simulink model "A4D_LQR_backup"  (R2016a)
settings: Solver=VariableStepAuto  StartTime=0.0  StopTime=10  RelTol=1e-3
undefined symbols (not defined in the file): A, B, C, K
settings Model: Creator=kumabhi  LastModifiedBy=kumabhi

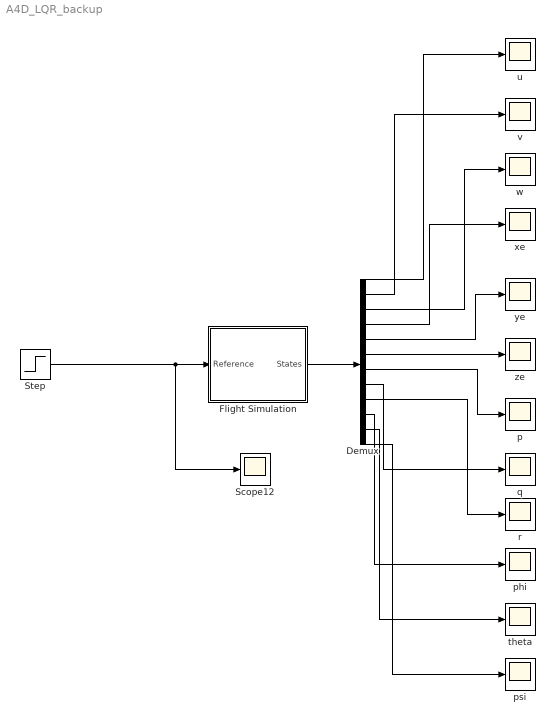
== system A4D_LQR_backup ==
  Demux : Demux  Outputs=12
  Flight Simulation : Subsystem
      mask Display: image('/home/kumabhi/Documents/Courses/Thesis/plane-icon-vector-.jpg');
  Scope12 : Scope
  Step : Step  After=1.0472  SampleTime=0
  p : Scope
  phi : Scope
  psi : Scope
  q : Scope
  r : Scope
  theta : Scope
  u : Scope
  v : Scope
  w : Scope
  xe : Scope
  ye : Scope
  ze : Scope
  wires:
  Step/1 -> Scope12/1, Flight Simulation/1(Reference)
  Flight Simulation/1(States) -> Demux/1
  Demux/1 -> u/1
  Demux/2 -> v/1
  Demux/3 -> w/1
  Demux/4 -> xe/1
  Demux/5 -> ye/1
  Demux/6 -> ze/1
  Demux/7 -> p/1
  Demux/8 -> q/1
  Demux/9 -> r/1
  Demux/10 -> phi/1
  Demux/11 -> theta/1
  Demux/12 -> psi/1

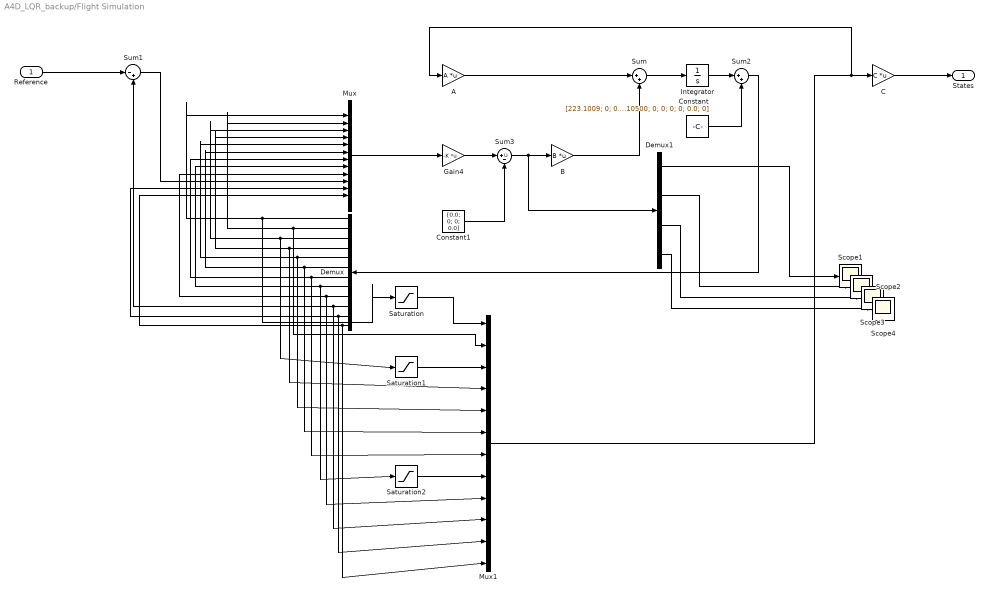
== system A4D_LQR_backup/Flight Simulation ==
  note: u
  Reference : Inport
  A : Gain  Gain=A  Multiplication=Matrix(K*u)
  B : Gain  Gain=B  Multiplication=Matrix(K*u)
  C : Gain  Gain=C  Multiplication=Matrix(K*u)
  Constant : Constant  Value=[223.1009; 0; 0.01; 0; 0; 10500; 0; 0; 0; 0; 0.0; 0]
  Constant1 : Constant  Value=[0.0; 0; 0; 0.0]
  Demux : Demux  Outputs=12
  Demux1 : Demux
  Gain4 : Gain  Gain=-K  Multiplication=Matrix(K*u)
  Integrator : Integrator
  Mux : Mux  Inputs=12
  Mux1 : Mux  Inputs=12
  Saturation : Saturate  UpperLimit=1000  LowerLimit=0
  Saturation1 : Saturate  UpperLimit=10  LowerLimit=0
  Saturation2 : Saturate  UpperLimit=100  LowerLimit=-100
  Scope{1..4} (4 alike) : Scope
  Sum : Sum  Inputs=|++
  Sum1 : Sum  Inputs=|-+
  Sum2 : Sum  Inputs=|++
  Sum3 : Sum  Inputs=|+-
  States : Outport
  wires:
  Reference/1 -> Sum1/1
  B/1 -> Sum/2
  C/1 -> States/1
  Demux/2 -> Mux/2, Mux1/2
  Demux/3 -> Saturation1/1, Mux/3
  Demux/4 -> Mux1/4, Mux/4
  Demux/5 -> Mux1/5, Mux/5
  Demux/6 -> Mux1/6, Mux/6
  Demux/7 -> Mux1/7, Mux/7
  Demux/8 -> Saturation2/1, Mux/8
  Demux/9 -> Mux1/9, Mux/9
  Mux/1 -> Gain4/1
  Demux/12 -> Mux1/12, Mux/12
  Demux1/1 -> Scope1/1
  Demux1/2 -> Scope2/1
  Demux1/3 -> Scope3/1
  Demux1/4 -> Scope4/1
  Demux/10 -> Mux1/10, Sum1/2
  Sum1/1 -> Mux/10
  Demux/1 -> Saturation/1, Mux/1
  A/1 -> Sum/1
  Sum/1 -> Integrator/1
  Integrator/1 -> Sum2/1
  Constant/1 -> Sum2/2
  Constant1/1 -> Sum3/2
  Gain4/1 -> Sum3/1
  Sum3/1 -> Demux1/1, B/1
  Saturation/1 -> Mux1/1
  Mux1/1 -> A/1, C/1
  Sum2/1 -> Demux/1
  Saturation1/1 -> Mux1/3
  Demux/11 -> Mux1/11, Mux/11
  Saturation2/1 -> Mux1/8
